simulink model "smib_IO"  (R2016a)
settings: Solver=VariableStepAuto  SolverMode=SingleTasking  StartTime=0.0  StopTime=10.0  RelTol=1e-3
undefined symbols (not defined in the file or in its folder): ExpandSmachs, j, machine_base_mva, s_D, s_delta, s_Edd, s_Efd, s_Eqd, s_H, s_Ka, s_Psi2q, s_Psild, s_Rgov, s_Rs, s_Ta, s_Tdod, s_Tdodd, s_Tg, s_Tm, s_Tqod, s_Tqodd, s_Vref, s_wb, s_ws, s_xd, s_xdd, s_xddd, s_xls, s_xq, s_xqd, s_xqdd, SelectSmachs, system_base_mva, Vinf, Zline
settings Model: Creator=lenovo  LastModifiedBy=EBUKA
settings DataIOCC: ReturnWorkspaceOutputs=on
settings DebuggingCC: SFUnexpectedBacktrackingDiag=error  SFNoUnconditionalDefaultTransitionDiag=error
settings SFSimCC: SimUseLocalCustomCode=on
settings RTWCC: RTWUseLocalCustomCode=on
settings GRTTargetCC: TargetLangStandard=C99 (ISO)  GeneratePreprocessorConditionals=Use local settings
settings ConfigComp: CovMetricSettings=dwe  CovHtmlReporting=off  CovSaveCumulativeToWorkspaceVar=off  CovSaveSingleToWorkspaceVar=off  CovExternalEMLEnable=on

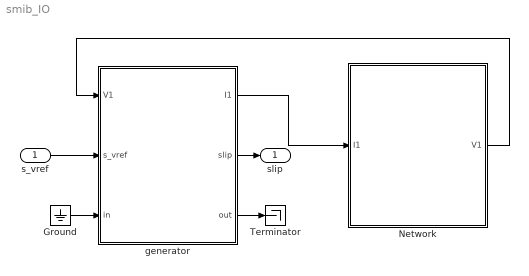
== system smib_IO ==
  s_vref : Inport
  Ground : Ground
  Network : Subsystem
  Terminator : Terminator
  generator : Subsystem
  slip : Outport
  wires:
  generator/1(I1) -> Network/1(I1)
  Network/1(V1) -> generator/1(V1)
  s_vref/1 -> generator/2(s_vref)
  generator/2(slip) -> slip/1
  generator/3(out) -> Terminator/1
  Ground/1 -> generator/3(in)

== system smib_IO/Network ==
  I1 : Inport
  Constant : Constant  Value=Vinf
  Gain : Gain  Gain=Zline  Multiplication=Matrix(K*u)
  Sum : Sum  Inputs=|++
  V1 : Outport
  wires:
  Gain/1 -> Sum/1
  I1/1 -> Gain/1
  Sum/1 -> V1/1
  Constant/1 -> Sum/2

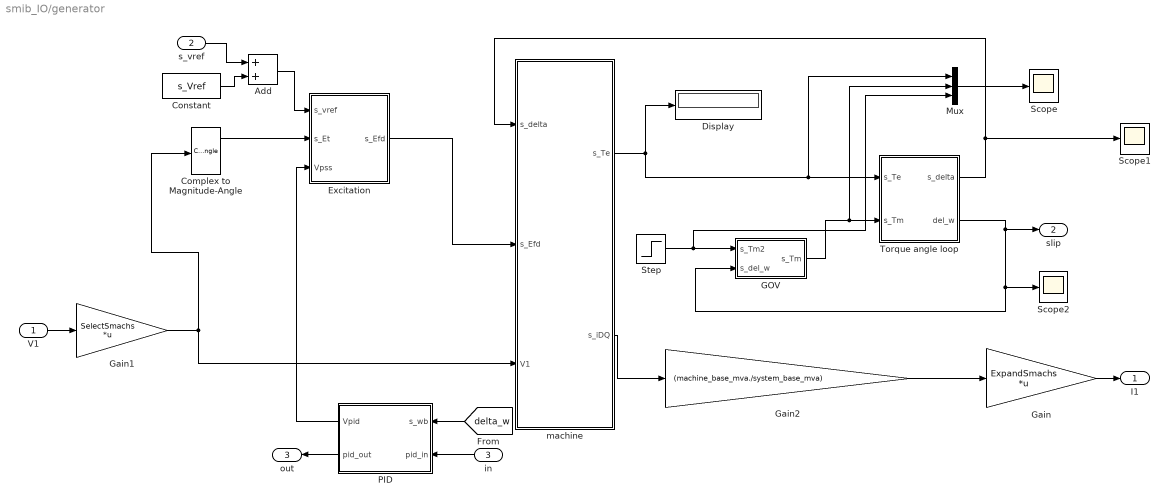
== system smib_IO/generator ==
  V1 : Inport
  s_vref : Inport  Port=2
  in : Inport  Port=3
  Add : Sum
  Complex to Magnitude-Angle : ComplexToMagnitudeAngle
  Constant : Constant  Value=s_Vref
  Display : Display
  Excitation : Subsystem
  GOV : Subsystem
  Gain : Gain  Gain=ExpandSmachs  Multiplication=Matrix(K*u)
  Gain1 : Gain  Gain=SelectSmachs  Multiplication=Matrix(K*u)
  Gain2 : Gain  Gain=(machine_base_mva./system_base_mva)
  Mux : Mux  Inputs=3
  PID : Subsystem
  Scope : Scope
  Scope1 : Scope
  Scope2 : Scope
  Step : Step  Before=s_Tm  After=(s_Tm)+0.007792  SampleTime=0
  Torque angle loop : Subsystem
  machine : Subsystem
  I1 : Outport
  slip : Outport  Port=2
  out : Outport  Port=3
  wires:
  machine/1(s_Te) -> Display/1, Mux/1, Torque angle loop/1(s_Te)
  V1/1 -> Gain1/1
  Gain1/1 -> machine/3(V1), Complex to Magnitude-Angle/1
  Complex to Magnitude-Angle/1 -> Excitation/2(s_Et)
  Gain/1 -> I1/1
  Excitation/1(s_Efd) -> machine/2(s_Efd)
  GOV/1(s_Tm) -> Mux/2, Torque angle loop/2(s_Tm)
  Torque angle loop/2(del_w) -> slip/1, Scope2/1, GOV/2(s_del_w)
  Add/1 -> Excitation/1(s_vref)
  s_vref/1 -> Add/1
  Constant/1 -> Add/2
  Torque angle loop/1("s_delta ") -> machine/1("s_delta "), Scope1/1
  Mux/1 -> Scope/1
  machine/2(s_iDQ) -> Gain2/1
  Gain2/1 -> Gain/1
  Step/1 -> Mux/3, GOV/1(s_Tm2)
  [delta_w] -> PID/1(s_wb)
  in/1 -> PID/2(pid_in)
  PID/1(Vpid) -> Excitation/3(Vpss)
  PID/2(pid_out) -> out/1

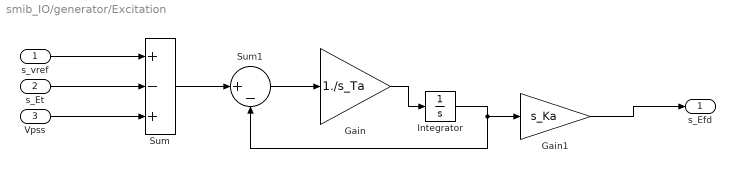
== system smib_IO/generator/Excitation ==
  s_vref : Inport
  s_Et : Inport  Port=2
  Vpss : Inport  Port=3
  Gain : Gain  Gain=1./s_Ta
  Gain1 : Gain  Gain=s_Ka
  Integrator : Integrator  InitialCondition=s_Efd./s_Ka
  Sum : Sum  Inputs=+-+
  Sum1 : Sum  Inputs=|+-
  s_Efd : Outport
  wires:
  s_vref/1 -> Sum/1
  s_Et/1 -> Sum/2
  Sum/1 -> Sum1/1
  Sum1/1 -> Gain/1
  Gain/1 -> Integrator/1
  Integrator/1 -> Sum1/2, Gain1/1
  Gain1/1 -> s_Efd/1
  Vpss/1 -> Sum/3

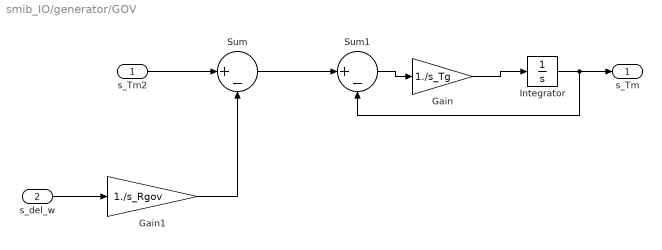
== system smib_IO/generator/GOV ==
  s_Tm2 : Inport
  s_del_w : Inport  Port=2
  Gain : Gain  Gain=1./s_Tg
  Gain1 : Gain  Gain=1./s_Rgov
  Integrator : Integrator  InitialCondition=s_Tm
  Sum : Sum  Inputs=|+-
  Sum1 : Sum  Inputs=|+-
  s_Tm : Outport
  wires:
  s_Tm2/1 -> Sum/1
  s_del_w/1 -> Gain1/1
  Sum/1 -> Sum1/1
  Sum1/1 -> Gain/1
  Gain/1 -> Integrator/1
  Integrator/1 -> Sum1/2, s_Tm/1
  Gain1/1 -> Sum/2

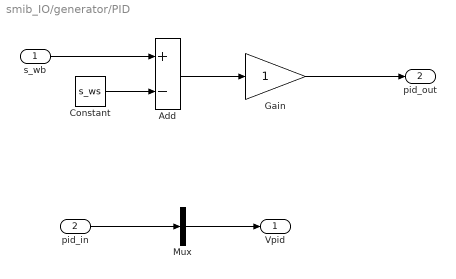
== system smib_IO/generator/PID ==
  s_wb : Inport
  pid_in : Inport  Port=2
  Add : Sum  Inputs=+-
  Constant : Constant  Value=s_ws
  Gain : Gain
  Mux : Mux  Inputs=1
  Vpid : Outport
  pid_out : Outport  Port=2
  wires:
  pid_in/1 -> Mux/1
  Mux/1 -> Vpid/1
  s_wb/1 -> Add/1
  Add/1 -> Gain/1
  Gain/1 -> pid_out/1
  Constant/1 -> Add/2

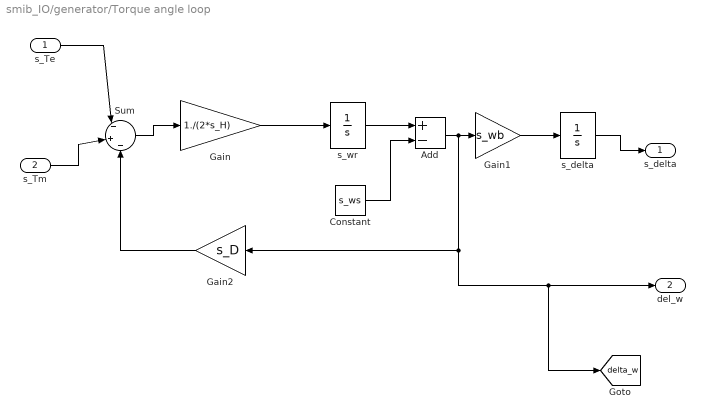
== system smib_IO/generator/Torque angle loop ==
  s_Te : Inport
  s_Tm : Inport  Port=2
  Add : Sum  Inputs=+-
  Constant : Constant  Value=s_ws
  Gain : Gain  Gain=1./(2*s_H)
  Gain1 : Gain  Gain=s_wb
  Gain2 : Gain  Gain=s_D
  Sum : Sum  Inputs=|-|+|-
  s_delta : Integrator  InitialCondition=s_delta
  s_wr : Integrator  InitialCondition=s_ws
  "s_delta " : Outport
  del_w : Outport  Port=2
  tag scope: delta_w=global
  wires:
  s_Tm/1 -> Sum/2
  Gain/1 -> s_wr/1
  s_delta/1 -> "s_delta "/1
  Constant/1 -> Add/2
  Sum/1 -> Gain/1
  s_wr/1 -> Add/1
  Gain1/1 -> s_delta/1
  Gain2/1 -> Sum/3
  Add/1 -> [delta_w], del_w/1, Gain2/1, Gain1/1
  s_Te/1 -> Sum/1

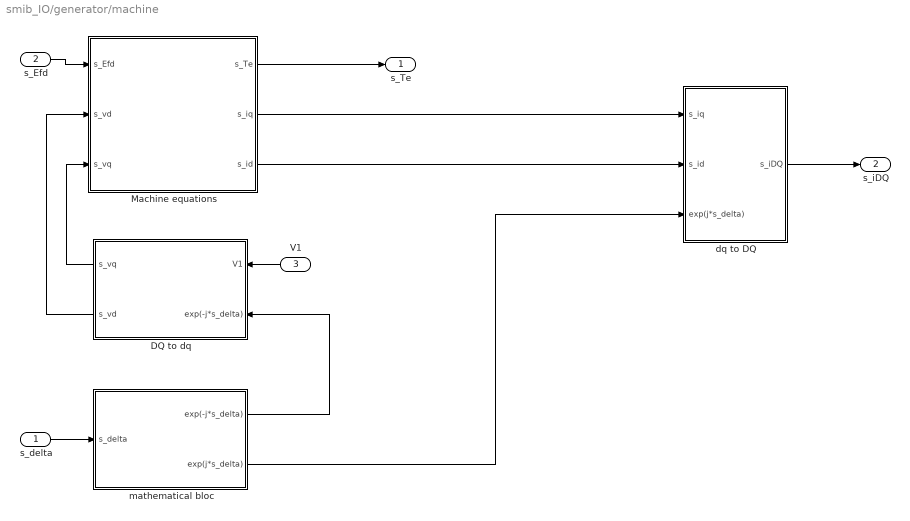
== system smib_IO/generator/machine ==
  "s_delta " : Inport
  s_Efd : Inport  Port=2
  V1 : Inport  Port=3
  DQ to dq : Subsystem
  Machine equations : Subsystem
  dq to DQ : Subsystem
  mathematical bloc : Subsystem
  s_Te : Outport
  s_iDQ : Outport  Port=2
  wires:
  "s_delta "/1 -> mathematical bloc/1("s_delta ")
  Machine equations/1(s_Te) -> s_Te/1
  s_Efd/1 -> Machine equations/1(s_Efd)
  V1/1 -> DQ to dq/1(V1)
  DQ to dq/1(s_vq) -> Machine equations/3(s_vq)
  DQ to dq/2(s_vd) -> Machine equations/2(s_vd)
  mathematical bloc/1(exp(-j*s_delta)) -> DQ to dq/2("exp(-j*s_delta) ")
  mathematical bloc/2(exp(j*s_delta)) -> dq to DQ/3(exp(j*s_delta))
  Machine equations/2(s_iq) -> dq to DQ/1(s_iq)
  Machine equations/3(s_id) -> dq to DQ/2(s_id)
  dq to DQ/1(s_iDQ) -> s_iDQ/1

== system smib_IO/generator/machine/DQ to dq ==
  V1 : Inport
  "exp(-j*s_delta) " : Inport  Port=2
  Complex to Real-Imag : ComplexToRealImag
  Product : Product
  s_vq : Outport
  s_vd : Outport  Port=2
  wires:
  "exp(-j*s_delta) "/1 -> Product/2
  V1/1 -> Product/1
  Product/1 -> Complex to Real-Imag/1
  Complex to Real-Imag/1 -> s_vq/1
  Complex to Real-Imag/2 -> s_vd/1

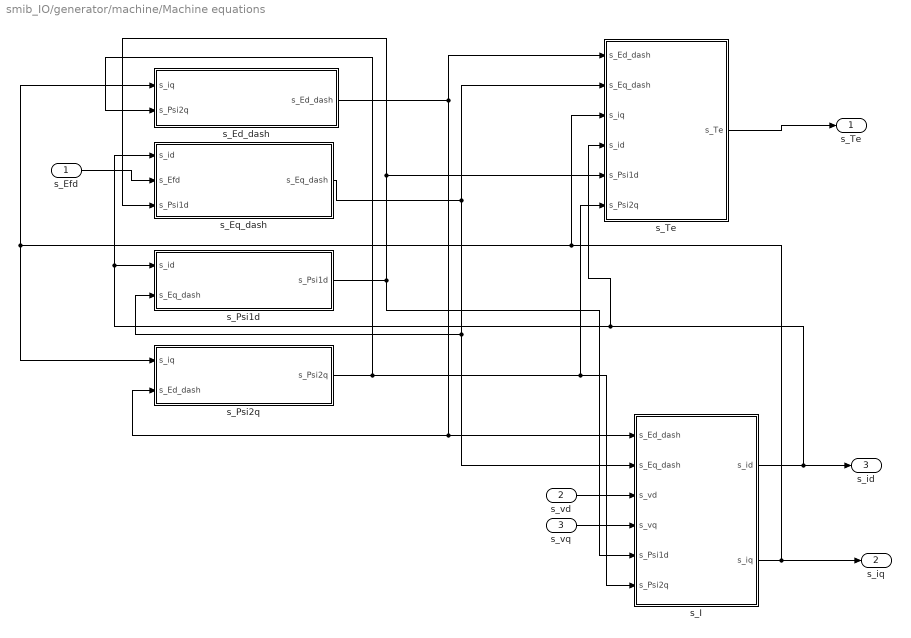
== system smib_IO/generator/machine/Machine equations ==
  s_Efd : Inport
  s_vd : Inport  Port=2
  s_vq : Inport  Port=3
  s_Ed_dash : Subsystem
  s_Eq_dash : Subsystem
  s_I : Subsystem
  s_Psi1d : Subsystem
  s_Psi2q : Subsystem
  "s_Te " : Subsystem
  s_Te : Outport
  s_iq : Outport  Port=2
  s_id : Outport  Port=3
  wires:
  s_Efd/1 -> s_Eq_dash/2(s_Efd)
  s_vd/1 -> s_I/3(s_vd)
  s_vq/1 -> s_I/4(s_vq)
  s_I/1(s_id) -> "s_Te "/4(s_id), s_Eq_dash/1(s_id), s_Psi1d/1(s_id), s_id/1
  s_I/2(s_iq) -> s_iq/1, "s_Te "/3(s_iq), s_Psi2q/1(s_iq), s_Ed_dash/1(s_iq)
  "s_Te "/1(s_Te) -> s_Te/1
  s_Ed_dash/1("s_Ed_dash ") -> "s_Te "/1("s_Ed_dash "), s_Psi2q/2("s_Ed_dash    "), s_I/1("s_Ed_dash  ")
  s_Eq_dash/1(s_Eq_dash) -> "s_Te "/2("s_Eq_dash "), s_I/2(s_Eq_dash), s_Psi1d/2(s_Eq_dash)
  s_Psi1d/1(s_Psi1d) -> s_I/5(s_Psi1d), "s_Te "/5(s_Psi1d), s_Eq_dash/3(s_Psi1d)
  s_Psi2q/1(s_Psi2q) -> "s_Te "/6(s_Psi2q), s_I/6(s_Psi2q), s_Ed_dash/2(s_Psi2q)

== system smib_IO/generator/machine/dq to DQ ==
  s_iq : Inport
  s_id : Inport  Port=2
  exp(j*s_delta) : Inport  Port=3
  Product : Product
  Real-Imag to Complex : RealImagToComplex
  s_iDQ : Outport
  wires:
  s_iq/1 -> Real-Imag to Complex/1
  s_id/1 -> Real-Imag to Complex/2
  Real-Imag to Complex/1 -> Product/1
  exp(j*s_delta)/1 -> Product/2
  Product/1 -> s_iDQ/1

== system smib_IO/generator/machine/mathematical bloc ==
  "s_delta " : Inport
  Gain : Gain  Gain=-j
  Gain1 : Gain  Gain=j
  Math Function : Math  SaturateOnIntegerOverflow=on
  Math Function1 : Math  SaturateOnIntegerOverflow=on
  exp(-j*s_delta) : Outport
  exp(j*s_delta) : Outport  Port=2
  wires:
  Gain/1 -> Math Function/1
  Math Function/1 -> exp(-j*s_delta)/1
  "s_delta "/1 -> Gain1/1, Gain/1
  Gain1/1 -> Math Function1/1
  Math Function1/1 -> exp(j*s_delta)/1

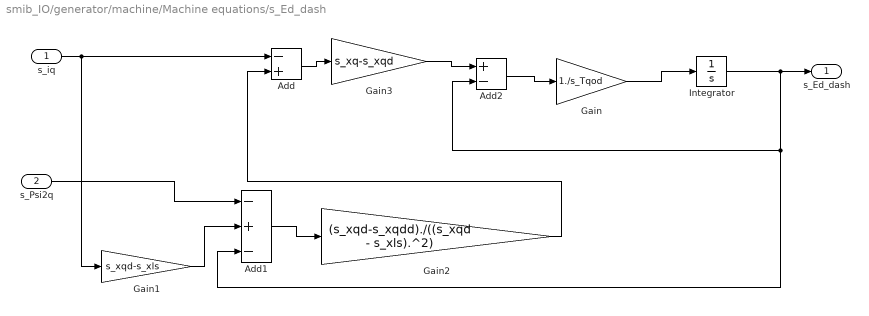
== system smib_IO/generator/machine/Machine equations/s_Ed_dash ==
  s_iq : Inport
  s_Psi2q : Inport  Port=2
  Add : Sum  Inputs=-+
  Add1 : Sum  Inputs=-+-
  Add2 : Sum  Inputs=+-
  Gain : Gain  Gain=1./s_Tqod
  Gain1 : Gain  Gain=s_xqd-s_xls
  Gain2 : Gain  Gain=(s_xqd-s_xqdd)./((s_xqd - s_xls).^2)
  Gain3 : Gain  Gain=s_xq-s_xqd
  Integrator : Integrator  InitialCondition=s_Edd
  "s_Ed_dash " : Outport
  wires:
  Add1/1 -> Gain2/1
  Gain/1 -> Integrator/1
  Gain1/1 -> Add1/2
  Gain2/1 -> Add/2
  Integrator/1 -> Add1/3, Add2/2, "s_Ed_dash "/1
  Add/1 -> Gain3/1
  s_iq/1 -> Add/1, Gain1/1
  s_Psi2q/1 -> Add1/1
  Gain3/1 -> Add2/1
  Add2/1 -> Gain/1

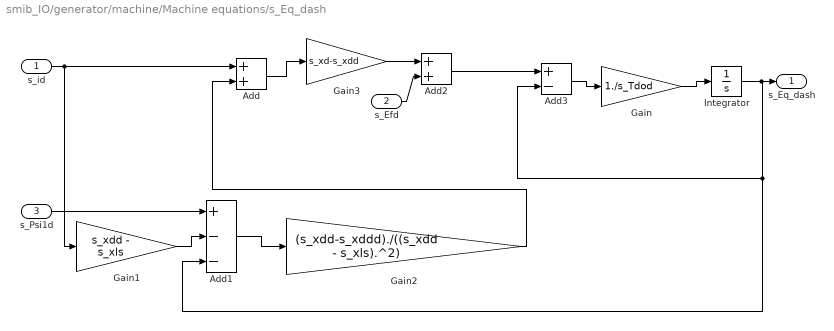
== system smib_IO/generator/machine/Machine equations/s_Eq_dash ==
  s_id : Inport
  s_Efd : Inport  Port=2
  s_Psi1d : Inport  Port=3
  Add : Sum
  Add1 : Sum  Inputs=+--
  Add2 : Sum
  Add3 : Sum  Inputs=+-
  Gain : Gain  Gain=1./s_Tdod
  Gain1 : Gain  Gain=s_xdd - s_xls
  Gain2 : Gain  Gain=(s_xdd-s_xddd)./((s_xdd - s_xls).^2)
  Gain3 : Gain  Gain=s_xd-s_xdd
  Integrator : Integrator  InitialCondition=s_Eqd
  s_Eq_dash : Outport
  wires:
  Add1/1 -> Gain2/1
  Gain/1 -> Integrator/1
  Gain1/1 -> Add1/2
  Gain2/1 -> Add/2
  Integrator/1 -> s_Eq_dash/1, Add1/3, Add3/2
  Add/1 -> Gain3/1
  s_id/1 -> Add/1, Gain1/1
  s_Psi1d/1 -> Add1/1
  s_Efd/1 -> Add2/2
  Gain3/1 -> Add2/1
  Add2/1 -> Add3/1
  Add3/1 -> Gain/1

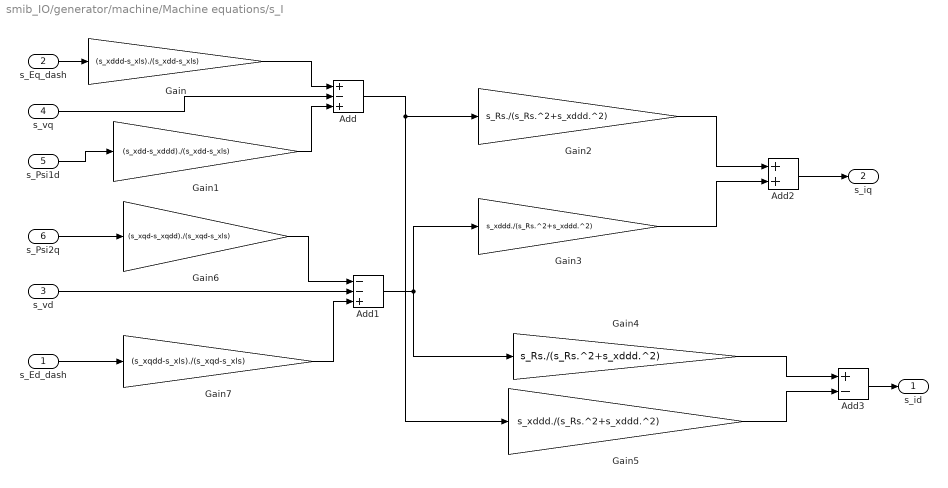
== system smib_IO/generator/machine/Machine equations/s_I ==
  "s_Ed_dash  " : Inport
  s_Eq_dash : Inport  Port=2
  s_vd : Inport  Port=3
  s_vq : Inport  Port=4
  s_Psi1d : Inport  Port=5
  s_Psi2q : Inport  Port=6
  Add : Sum  Inputs=+-+
  Add1 : Sum  Inputs=--+
  Add2 : Sum
  Add3 : Sum  Inputs=+-
  Gain : Gain  Gain=(s_xddd-s_xls)./(s_xdd-s_xls)
  Gain1 : Gain  Gain=(s_xdd-s_xddd)./(s_xdd-s_xls)
  Gain2 : Gain  Gain=s_Rs./(s_Rs.^2+s_xddd.^2)
  Gain3 : Gain  Gain=s_xddd./(s_Rs.^2+s_xddd.^2)
  Gain4 : Gain  Gain=s_Rs./(s_Rs.^2+s_xddd.^2)
  Gain5 : Gain  Gain=s_xddd./(s_Rs.^2+s_xddd.^2)
  Gain6 : Gain  Gain=(s_xqd-s_xqdd)./(s_xqd-s_xls)
  Gain7 : Gain  Gain=(s_xqdd-s_xls)./(s_xqd-s_xls)
  s_id : Outport
  s_iq : Outport  Port=2
  wires:
  s_Eq_dash/1 -> Gain/1
  Gain/1 -> Add/1
  s_vq/1 -> Add/2
  s_Psi1d/1 -> Gain1/1
  Gain1/1 -> Add/3
  Add/1 -> Gain5/1, Gain2/1
  Gain2/1 -> Add2/1
  Add2/1 -> s_iq/1
  Add1/1 -> Gain3/1, Gain4/1
  Gain3/1 -> Add2/2
  Add3/1 -> s_id/1
  Gain4/1 -> Add3/1
  Gain5/1 -> Add3/2
  s_Psi2q/1 -> Gain6/1
  Gain6/1 -> Add1/1
  s_vd/1 -> Add1/2
  Gain7/1 -> Add1/3
  "s_Ed_dash  "/1 -> Gain7/1

== system smib_IO/generator/machine/Machine equations/s_Psi1d ==
  s_id : Inport
  s_Eq_dash : Inport  Port=2
  Add : Sum  Inputs=++-
  Gain : Gain  Gain=s_xdd-s_xls
  Gain1 : Gain  Gain=1./s_Tdodd
  Integrator : Integrator  InitialCondition=s_Psild
  s_Psi1d : Outport
  wires:
  Integrator/1 -> Add/3, s_Psi1d/1
  Gain1/1 -> Integrator/1
  Add/1 -> Gain1/1
  s_id/1 -> Gain/1
  Gain/1 -> Add/1
  s_Eq_dash/1 -> Add/2

== system smib_IO/generator/machine/Machine equations/s_Psi2q ==
  s_iq : Inport
  "s_Ed_dash    " : Inport  Port=2
  Add : Sum  Inputs=+--
  Gain : Gain  Gain=s_xqd-s_xls
  Gain1 : Gain  Gain=1./s_Tqodd
  Integrator : Integrator  InitialCondition=s_Psi2q
  s_Psi2q : Outport
  wires:
  Gain/1 -> Add/1
  "s_Ed_dash    "/1 -> Add/2
  Gain1/1 -> Integrator/1
  s_iq/1 -> Gain/1
  Add/1 -> Gain1/1
  Integrator/1 -> s_Psi2q/1, Add/3

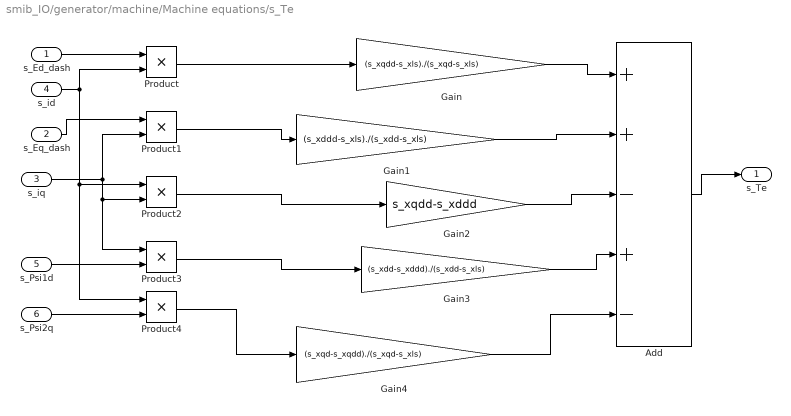
== system smib_IO/generator/machine/Machine equations/s_Te  ==
  "s_Ed_dash " : Inport
  "s_Eq_dash " : Inport  Port=2
  s_iq : Inport  Port=3
  s_id : Inport  Port=4
  s_Psi1d : Inport  Port=5
  s_Psi2q : Inport  Port=6
  Add : Sum  Inputs=++-+-
  Gain : Gain  Gain=(s_xqdd-s_xls)./(s_xqd-s_xls)
  Gain1 : Gain  Gain=(s_xddd-s_xls)./(s_xdd-s_xls)
  Gain2 : Gain  Gain=s_xqdd-s_xddd
  Gain3 : Gain  Gain=(s_xdd-s_xddd)./(s_xdd-s_xls)
  Gain4 : Gain  Gain=(s_xqd-s_xqdd)./(s_xqd-s_xls)
  Product{,1..4} (5 alike) : Product
  s_Te : Outport
  wires:
  "s_Ed_dash "/1 -> Product/1
  s_id/1 -> Product4/1, Product2/1, Product/2
  "s_Eq_dash "/1 -> Product1/1
  s_iq/1 -> Product1/2, Product2/2, Product3/1
  s_Psi1d/1 -> Product3/2
  s_Psi2q/1 -> Product4/2
  Product/1 -> Gain/1
  Product1/1 -> Gain1/1
  Product2/1 -> Gain2/1
  Product3/1 -> Gain3/1
  Product4/1 -> Gain4/1
  Add/1 -> s_Te/1
  Gain/1 -> Add/1
  Gain1/1 -> Add/2
  Gain2/1 -> Add/3
  Gain3/1 -> Add/4
  Gain4/1 -> Add/5
